simulink model "hamowanie_samolotu"  (R2021b)
settings: Solver=VariableStepAuto  StartTime=0.0  StopTime=10.0  RelTol=1e-3
values from neighbouring files (symbols this model uses):
  h = 42    [mlab.m]
  k1 = 54700    [mlab.m]
  k2 = 303600    [mlab.m]
  m1 = 14000    [mlab.m]
  m2 = 450.28    [mlab.m]
  m3 = 200    [mlab.m]
settings Model: Creator=jpawl  LastModifiedBy=jpawl

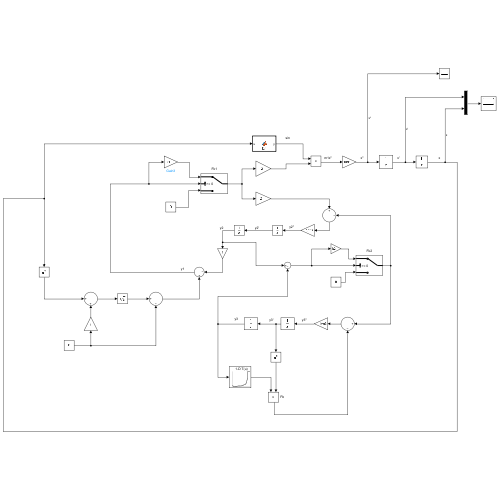
[thumbnail: Simulink's stored preview of the top-level diagram]
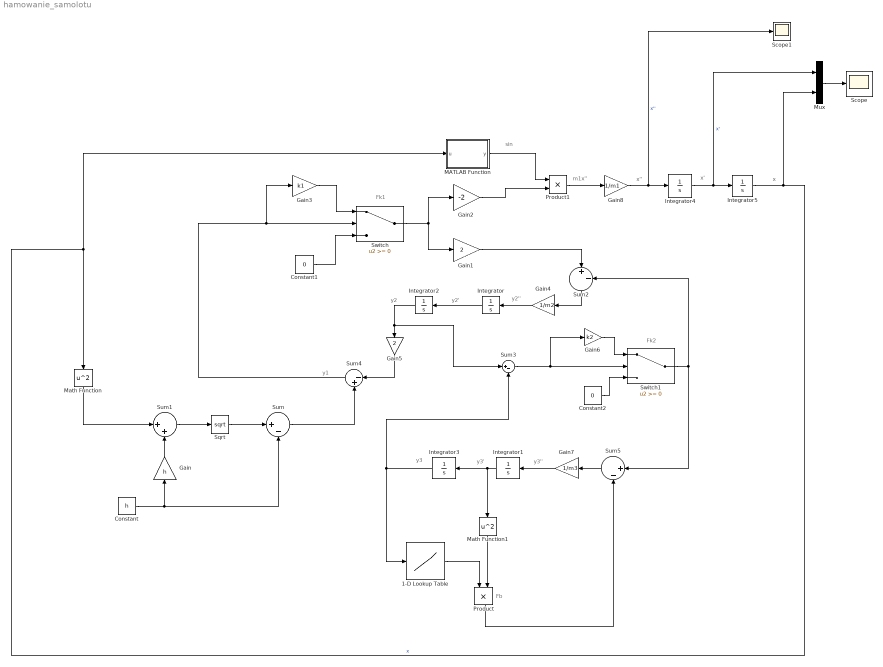
== system hamowanie_samolotu ==
  note: Fb
  note: x
  note: m1x''
  note: sin
  note: x'
  note: x''
  note: y3
  note: y3'
  note: y3''
  note: y1
  note: y2
  note: y2'
  note: y2''
  note: Fk2
  note: Fk1
  1-D Lookup Table : Lookup_n-D  NumberOfTableDimensions=1  BreakpointsForDimension1=[0, 10, 20, 30, 40, 50, 60, 70, 80, 90, 94, 98, 102, 104, 107, 120]  Table=[833, 400, 160, 320, 520, 520, 660, 830, 1070, 1600, 2100, 2800, 4100, 5000, 9000, 9000]  InternalRulePriority=Speed  RndMeth=Simplest  InputSameDT=on
  Constant : Constant  Value=h
  Constant1 : Constant  Value=0
  Constant2 : Constant  Value=0
  Gain : Gain  Gain=h
  Gain1 : Gain  Gain=2
  Gain2 : Gain  Gain=-2
  Gain3 : Gain  Gain=k1
  Gain4 : Gain  Gain=1/m2
  Gain5 : Gain  Gain=2
  Gain6 : Gain  Gain=k2
  Gain7 : Gain  Gain=1/m3
  Gain8 : Gain  Gain=1/m1
  Integrator{,1..3,5} (5 alike) : Integrator
  Integrator4 : Integrator  InitialCondition=67
  MATLAB Function : MATLAB Function  TreatAsAtomicUnit=on
  Math Function : Math  Operator=square  SaturateOnIntegerOverflow=on
  Math Function1 : Math  Operator=square  SaturateOnIntegerOverflow=on
  Mux : Mux  Inputs=2
  Product : Product
  Product1 : Product
  Scope : Scope
  Scope1 : Scope
  Sqrt : Sqrt  SaturateOnIntegerOverflow=on
  Sum{,2..3,5} (4 alike) : Sum  Inputs=|+-
  Sum1 : Sum  Inputs=|++
  Sum4 : Sum  Inputs=|-+
  Switch : Switch
  Switch1 : Switch
  wires:
  Constant/1 -> Sum/2, Gain/1
  Gain/1 -> Sum1/2
  Sum1/1 -> Sqrt/1
  Sqrt/1 -> Sum/1
  Math Function/1 -> Sum1/1
  Switch/1 -> Gain2/1, Gain1/1
  Gain1/1 -> Sum2/1
  Switch1/1 -> Sum2/2, Sum5/1
  Gain3/1 -> Switch/1
  Constant1/1 -> Switch/3
  Sum2/1 -> Gain4/1
  Gain4/1 -> Integrator/1
  Integrator/1 -> Integrator2/1
  Integrator2/1 -> Gain5/1, Sum3/1
  Sum/1 -> Sum4/2
  Gain5/1 -> Sum4/1
  Sum4/1 -> Gain3/1, Switch/2
  Constant2/1 -> Switch1/3
  Gain6/1 -> Switch1/1
  Sum3/1 -> Gain6/1, Switch1/2
  Product/1 -> Sum5/2
  Sum5/1 -> Gain7/1
  Gain7/1 -> Integrator1/1
  Integrator1/1 -> Math Function1/1, Integrator3/1
  Integrator3/1 -> Sum3/2, 1-D Lookup Table/1
  Math Function1/1 -> Product/2
  1-D Lookup Table/1 -> Product/1
  Gain2/1 -> Product1/2
  MATLAB Function/1(y) -> Product1/1
  Product1/1 -> Gain8/1
  Gain8/1 -> Scope1/1, Integrator4/1  "x''"
  Integrator4/1 -> Mux/1, Integrator5/1  "x'"
  Integrator5/1 -> Mux/2, Math Function/1, MATLAB Function/1(u)  "x"
  Mux/1 -> Scope/1

== matlab function hamowanie_samolotu/MATLAB Function ==
  data: u input; y output
function y = fcn(u)
h = 42;
y = u/(sqrt(u^2 + h^2));
